simulink model "JenaFox_NCm"  (R2022a)
settings: Solver=VariableStepAuto  StartTime=0.0  StopTime=terminationConditions.stopTime  FixedStep=0.0001  MaxStep=solverParams.maxStep  RelTol=solverParams.relTol  AbsTol=solverParams.absTol
undefined symbols (not defined in the file): amplifier, c_coupling, d_coupling, g, GC, GM_h, IC, IC_v, motorHip, motorKnee, mu, offset, prop_const, smiData, terminationConditions, v, X, Y, Z
libraries: sm_lib x51, nesl_utility x46, simulink x23, simulink_extras x12, dspswit3 x2
(part 1 of 4)
settings Model: SimulationMode=accelerator  Creator=Work  LastModifiedBy=fesch
settings SolverCC: NumberNewtonIterations=2  ZeroCrossAlgorithm=Adaptive  AlgebraicLoopSolver=TrustRegion
settings DataIOCC: ExternalInput=JenaFox_NCm  FinalStateName=finalOP  SaveOperatingPoint=on  Refine=solverParams.refineFactor
settings DebuggingCC: IgnoredZcDiagnostic=none  UnconnectedInputMsg=warning  UnconnectedOutputMsg=warning  UnconnectedLineMsg=warning  SFMachineParentedDataDiag=warning  ArithmeticOperatorsInVariantConditions=warning
settings SFSimCC: SimUseLocalCustomCode=off  CustomCodeUndefinedFunction=UseInterfaceOnly
settings RTWCC: RTWUseLocalCustomCode=off  Toolchain=MinGW64 | gmake (64-bit Windows)  DLArmComputeVersion=19.05
settings ExplorerConfigSet: InternalSimMechanicsExplorerSettings="<ExplorerConfiguration><canonicalview>planar_xy</canonicalview><AnimationSetting><BasePlaybackSpeed>1.0</BasePlaybackSpeed><PlaybackSpeedFactor>0.25</PlaybackSpeedFactor></AnimationSetting><TilePanel><TileInfo><Tiles Columns=\"1\" Count=\"1\" Rows=\"1\"><Column Weight=\"1\"/><Row Weight=\"1\"/><Tile Height=\"1\" Width=\"1\" X=\"0\" Y=\"0\"/></Tiles></TileInfo><SceneInfo><SceneViewer><BGColor><R>1</R><G>1</G><B>1</B></BGColor><Camera><DoPerspective>on</DoPerspective><Position><X>0.0780946526691303905</X><Y>0.155519108041309417</Y><Z>0.5</Z></Position><Center><X>0.0780946526691303905</X><Y>0.155519108041309417</Y><Z>-0.5</Z></Center><Up><X>-9.313783918415811e-06</X><Y>0.999999999956626695</Y><Z>0</Z></Up><ViewLimDist>1</ViewLimDist><YLim>0.466307658154998583</YLim><XLim>0.934484284879756544</XLim></Camera></SceneViewer></SceneInfo></TilePanel><MechEditorPanel><Cameras><Camera><Id>Camera1</Id><Value><Name>Camera1</Name><NativeCamera><PositionTrackingFeature>JenaFox_model.Camera1.Frame1</PositionTrackingFeature><CenterTrackingFeature>JenaFox_model.Camera1.Frame1</CenterTrackingFeature><UpVectorTrackingFeature>JenaFox_model.Camera1.Frame1</UpVectorTrackingFeature><CenterTrackingOrigin>off</CenterTrackingOrigin><CenterTrackingDirection>-Z</CenterTrackingDirection><UpVectorTrackingDirection>+Y</UpVectorTrackingDirection></NativeCamera></Value></Camera></Cameras><GfxPanelCameraMap><MapElement CameraMLId=\"Camera1\" GfxPanelIndex=\"0\"/></GfxPanelCameraMap><VideoCreator><PlaybackSpeedRatio>0.25</PlaybackSpeedRatio><FrameRate>30</FrameRate><VideoFormat>Motion JPEG AVI</VideoFormat><FrameSize>auto</FrameSize></VideoCreator></MechEditorPanel></ExplorerConfiguration>"

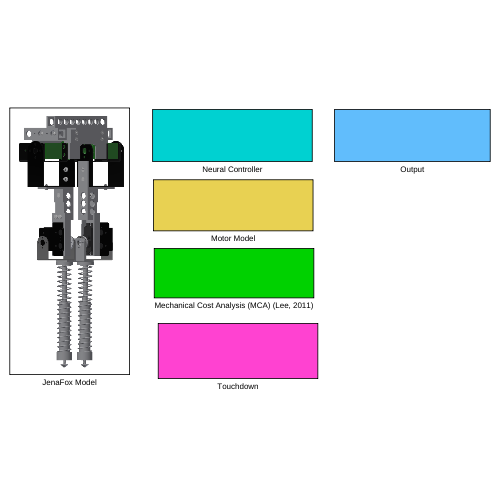
[thumbnail: Simulink's stored preview of the top-level diagram]
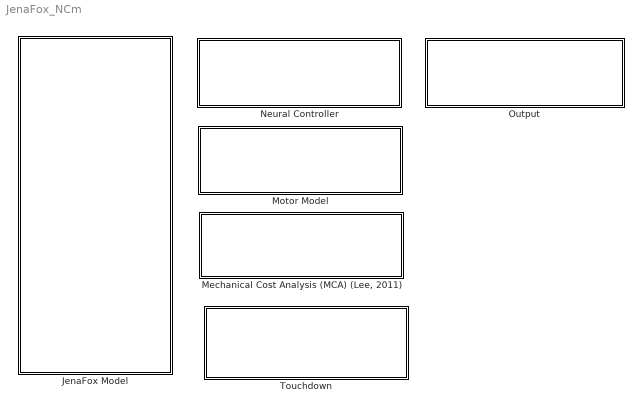
== system JenaFox_NCm ==
  JenaFox Model : Subsystem
      mask Display: image('$imagefile'); % Use "Edit Image" on toolstrip to change.
  "Mechanical Cost Analysis (MCA) (Lee, 2011)" : Subsystem
  Motor Model : Subsystem
  Neural Controller : Subsystem
  Output : Subsystem
  Touchdown : Subsystem

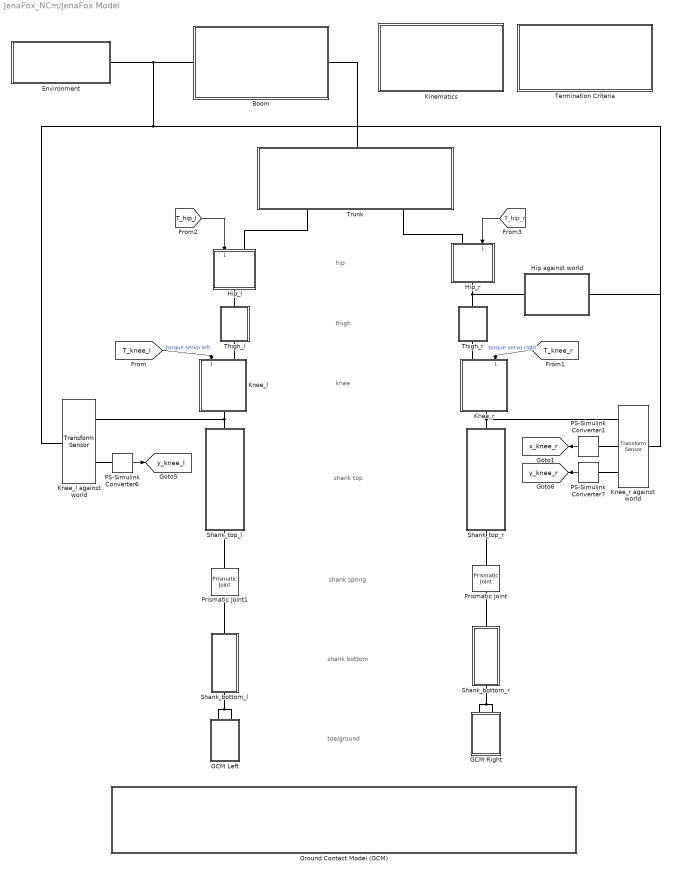
== system JenaFox_NCm/JenaFox Model ==
  note: hip
  note: thigh
  note: knee
  note: shank top
  note: shank spring
  note: shank bottom
  note: toe/ground
  Boom : Subsystem
  Environment : Subsystem
  GCM Left : Subsystem
      settings: PortSchema="{\"entries\":[{\"content\":{\"sides\":[{\"content\":{\"connectorIds\":[]},\"type\":\"ConnectorPlacement.EquallySpacedRectSide\",\"uuid\":\"717cb0e6-c62a-4e06-8591-18c3af15a403\"},{\"content\":{\"connectorIds\":[],\"side\":\"RIGHT\"},\"type\":\"ConnectorPlacement.EquallySpacedRectSide\",\"uuid\":\"b55d33af-557a-4e38-8805-fc673b8726f4\"},{\"content\":{\"connectorIds\":[\"LConn1\",\"LConn2\"],\"side\":\"TOP\"},\"type\":\"ConnectorPlacement.EquallySpacedRectSide\",\"uuid\":\"c2e40c4e-431e-4c5b-992c-f2657d397cd9\"}]},\"type\":\"ConnectorPlacement.EquallySpacedConnector\",\"uuid\":\"60787a51-cbf9-4fb7-a22c-83b01a92506b\"}],\"packageUris\":[\"http://schema.mathworks.com/mf0/Connector/R2020b\"],\"version\":\"1.0\"}"
  GCM Right : Subsystem
      settings: PortSchema="{\"entries\":[{\"content\":{\"sides\":[{\"content\":{\"connectorIds\":[]},\"type\":\"ConnectorPlacement.EquallySpacedRectSide\",\"uuid\":\"717cb0e6-c62a-4e06-8591-18c3af15a403\"},{\"content\":{\"connectorIds\":[],\"side\":\"RIGHT\"},\"type\":\"ConnectorPlacement.EquallySpacedRectSide\",\"uuid\":\"b55d33af-557a-4e38-8805-fc673b8726f4\"},{\"content\":{\"connectorIds\":[\"LConn1\",\"LConn2\"],\"side\":\"TOP\"},\"type\":\"ConnectorPlacement.EquallySpacedRectSide\",\"uuid\":\"c2e40c4e-431e-4c5b-992c-f2657d397cd9\"}]},\"type\":\"ConnectorPlacement.EquallySpacedConnector\",\"uuid\":\"60787a51-cbf9-4fb7-a22c-83b01a92506b\"}],\"packageUris\":[\"http://schema.mathworks.com/mf0/Connector/R2020b\"],\"version\":\"1.0\"}"
  Ground Contact Model (GCM) : Subsystem
  Hip against world : Subsystem
  Hip_l : Subsystem
  Hip_r : Subsystem
      settings: PortSchema="{\"entries\":[{\"content\":{\"sides\":[{\"content\":{\"connectorIds\":[\"LConn1\",\"In1\"]},\"type\":\"ConnectorPlacement.EquallySpacedRectSide\",\"uuid\":\"6727c252-b3e4-4702-a459-ab364fb8daee\"},{\"content\":{\"connectorIds\":[\"RConn1\"],\"side\":\"RIGHT\"},\"type\":\"ConnectorPlacement.EquallySpacedRectSide\",\"uuid\":\"d9cb8ba9-0a5e-46cb-8448-2d23ff2cf8a0\"},{\"content\":{\"connectorIds\":[],\"side\":\"TOP\"},\"type\":\"ConnectorPlacement.EquallySpacedRectSide\",\"uuid\":\"eb700dfb-5883-4c49-bb8c-e592edc073a0\"}]},\"type\":\"ConnectorPlacement.EquallySpacedConnector\",\"uuid\":\"4bb2fdc9-2c2e-463e-9c20-4381bcff8659\"}],\"packageUris\":[\"http://schema.mathworks.com/mf0/Connector/R2020b\"],\"version\":\"1.0\"}"
  Kinematics : Subsystem
  Knee_l : Subsystem
  Knee_l against world : sm_lib/Frames and Transforms/Transform Sensor  MeasurementFrame=World  SenseAngle=off  SenseAxis=off  SenseAngle1=off  SenseAngle2=off  SenseAngle3=off  SenseQ=off  SenseR=off  SenseOmegaX=off  SenseOmegaY=off  SenseOmegaZ=off  SenseOmega1=off  SenseOmega2=off  SenseOmega3=off  SenseQDot=off  SenseRDot=off  SenseAlphaX=off  SenseAlphaY=off  SenseAlphaZ=off  SenseAlpha1=off  SenseAlpha2=off  SenseAlpha3=off  SenseQDDot=off  SenseRDDot=off  SenseX=off  SenseY=on  SenseZ=off  SenseRad=off  SenseAzim=off  SenseDist=off  SenseInc=off  SenseXDot=off  SenseYDot=off  SenseZDot=off  SenseRadDot=off  SenseAzimDot=off  SenseDistDot=off  SenseIncDot=off  SenseXDDot=off  SenseYDDot=off  SenseZDDot=off  SenseRadDDot=off  SenseAzimDDot=off  SenseDistDDot=off  SenseIncDDot=off
  Knee_r : Subsystem
      settings: PortSchema="{\"entries\":[{\"content\":{\"sides\":[{\"content\":{\"connectorIds\":[\"LConn1\",\"In1\"]},\"type\":\"ConnectorPlacement.EquallySpacedRectSide\",\"uuid\":\"6727c252-b3e4-4702-a459-ab364fb8daee\"},{\"content\":{\"connectorIds\":[\"RConn1\"],\"side\":\"RIGHT\"},\"type\":\"ConnectorPlacement.EquallySpacedRectSide\",\"uuid\":\"d9cb8ba9-0a5e-46cb-8448-2d23ff2cf8a0\"},{\"content\":{\"connectorIds\":[],\"side\":\"TOP\"},\"type\":\"ConnectorPlacement.EquallySpacedRectSide\",\"uuid\":\"eb700dfb-5883-4c49-bb8c-e592edc073a0\"}]},\"type\":\"ConnectorPlacement.EquallySpacedConnector\",\"uuid\":\"4bb2fdc9-2c2e-463e-9c20-4381bcff8659\"}],\"packageUris\":[\"http://schema.mathworks.com/mf0/Connector/R2020b\"],\"version\":\"1.0\"}"
  Knee_r against world : sm_lib/Frames and Transforms/Transform Sensor  MeasurementFrame=World  SenseAngle=off  SenseAxis=off  SenseAngle1=off  SenseAngle2=off  SenseAngle3=off  SenseQ=off  SenseR=off  SenseOmegaX=off  SenseOmegaY=off  SenseOmegaZ=off  SenseOmega1=off  SenseOmega2=off  SenseOmega3=off  SenseQDot=off  SenseRDot=off  SenseAlphaX=off  SenseAlphaY=off  SenseAlphaZ=off  SenseAlpha1=off  SenseAlpha2=off  SenseAlpha3=off  SenseQDDot=off  SenseRDDot=off  SenseX=on  SenseY=on  SenseZ=off  SenseRad=off  SenseAzim=off  SenseDist=off  SenseInc=off  SenseXDot=off  SenseYDot=off  SenseZDot=off  SenseRadDot=off  SenseAzimDot=off  SenseDistDot=off  SenseIncDot=off  SenseXDDot=off  SenseYDDot=off  SenseZDDot=off  SenseRadDDot=off  SenseAzimDDot=off  SenseDistDDot=off  SenseIncDDot=off
  PS-Simulink Converter1 : nesl_utility/PS-Simulink Converter  PhysicalDomain=network_engine_domain  SubClassName=ps_output  LeftPortType=input  RightPortType=output  PseudoPeriodic=off  Frequencies=[]  VectorFormat=1-D array  Unit=1  AffineConversion=off
      settings: SourceProductBaseCode=SS,PW,VE
  PS-Simulink Converter6 : nesl_utility/PS-Simulink Converter  PhysicalDomain=network_engine_domain  SubClassName=ps_output  LeftPortType=input  RightPortType=output  PseudoPeriodic=off  Frequencies=[]  VectorFormat=1-D array  Unit=1  AffineConversion=off
      settings: SourceProductBaseCode=SS,PW,VE
  PS-Simulink Converter7 : nesl_utility/PS-Simulink Converter  PhysicalDomain=network_engine_domain  SubClassName=ps_output  LeftPortType=input  RightPortType=output  PseudoPeriodic=off  Frequencies=[]  VectorFormat=1-D array  Unit=1  AffineConversion=off
      settings: SourceProductBaseCode=SS,PW,VE
  Prismatic Joint : sm_lib/Joints/Prismatic Joint  JointMode=Normal  SenseConstraintForce=off  SenseConstraintForceX=off  SenseConstraintForceY=off  SenseConstraintForceZ=off  SenseConstraintTorque=off  SenseConstraintTorqueX=off  SenseConstraintTorqueY=off  SenseConstraintTorqueZ=off  SenseTotalForce=off  SenseTotalForceX=off  SenseTotalForceY=off  SenseTotalForceZ=off  SenseTotalTorque=off  SenseTotalTorqueX=off  SenseTotalTorqueY=off  SenseTotalTorqueZ=off  CompositeWrenchDir=FollowerOnBase  CompositeWrenchFrame=BaseFrame  EquilibriumPosition=0  EquilibriumPositionUnits=m  SpringStiffness=springAnkle.c_r  SpringStiffnessUnits=N/m  DampingCoefficient=damperAnkle.r  DampingCoefficientUnits=N/(m/s)  TorqueActuationMode=NoTorque  MotionActuationMode=ComputedMotion  SensePosition=off  SenseVelocity=off  SenseAcceleration=off  SenseTorqueForce=off  SenseLowerLimitTorqueForce=off  SenseUpperLimitTorqueForce=off  LowerLimitSpecify=off  LowerLimitBound=-1  LowerLimitBoundUnits=m  LowerLimitStiffness=1e6  LowerLimitStiffnessUnits=N/m  LowerLimitDamping=1e3  LowerLimitDampingUnits=N/(m/s)  LowerLimitTransitionRegionWidth=1e-4  LowerLimitTransitionRegionWidthUnits=m  UpperLimitSpecify=on  UpperLimitBound=0  UpperLimitBoundUnits=m  UpperLimitStiffness=1e6  UpperLimitStiffnessUnits=N/m  UpperLimitDamping=1e3  UpperLimitDampingUnits=N/(m/s)  UpperLimitTransitionRegionWidth=1e-4  UpperLimitTransitionRegionWidthUnits=m  PositionTargetSpecify=off  PositionTargetPriority=High  PositionTargetValue=0  PositionTargetValueUnits=m  VelocityTargetSpecify=off  VelocityTargetPriority=High  VelocityTargetValue=0  VelocityTargetValueUnits=m/s
  Prismatic Joint1 : sm_lib/Joints/Prismatic Joint  JointMode=Normal  SenseConstraintForce=off  SenseConstraintForceX=off  SenseConstraintForceY=off  SenseConstraintForceZ=off  SenseConstraintTorque=off  SenseConstraintTorqueX=off  SenseConstraintTorqueY=off  SenseConstraintTorqueZ=off  SenseTotalForce=off  SenseTotalForceX=off  SenseTotalForceY=off  SenseTotalForceZ=off  SenseTotalTorque=off  SenseTotalTorqueX=off  SenseTotalTorqueY=off  SenseTotalTorqueZ=off  CompositeWrenchDir=FollowerOnBase  CompositeWrenchFrame=BaseFrame  EquilibriumPosition=0  EquilibriumPositionUnits=m  SpringStiffness=springAnkle.c_l  SpringStiffnessUnits=N/m  DampingCoefficient=damperAnkle.l  DampingCoefficientUnits=N/(m/s)  TorqueActuationMode=NoTorque  MotionActuationMode=ComputedMotion  SensePosition=off  SenseVelocity=off  SenseAcceleration=off  SenseTorqueForce=off  SenseLowerLimitTorqueForce=off  SenseUpperLimitTorqueForce=off  LowerLimitSpecify=off  LowerLimitBound=-1  LowerLimitBoundUnits=m  LowerLimitStiffness=1e6  LowerLimitStiffnessUnits=N/m  LowerLimitDamping=1e3  LowerLimitDampingUnits=N/(m/s)  LowerLimitTransitionRegionWidth=1e-4  LowerLimitTransitionRegionWidthUnits=m  UpperLimitSpecify=on  UpperLimitBound=0  UpperLimitBoundUnits=m  UpperLimitStiffness=1e6  UpperLimitStiffnessUnits=N/m  UpperLimitDamping=1e3  UpperLimitDampingUnits=N/(m/s)  UpperLimitTransitionRegionWidth=1e-4  UpperLimitTransitionRegionWidthUnits=m  PositionTargetSpecify=off  PositionTargetPriority=High  PositionTargetValue=0  PositionTargetValueUnits=m  VelocityTargetSpecify=off  VelocityTargetPriority=High  VelocityTargetValue=0  VelocityTargetValueUnits=m/s
  Shank_bottom_l : Subsystem
  Shank_bottom_r : Subsystem
  Shank_top_l : Subsystem
  Shank_top_r : Subsystem
  Termination Criteria : Subsystem
  Thigh_l : Subsystem
  Thigh_r : Subsystem
  Trunk : Subsystem
  tag scope: x_knee_r=global, y_knee_l=global, y_knee_r=global
  wires:
  [T_knee_l] -> Knee_l/1(Left torque)  "torque servo left"
  [T_knee_r] -> Knee_r/1(Right torque)  "torque servo right"
  [T_hip_l] -> Hip_l/1(Left torque)
  [T_hip_r] -> Hip_r/1(Right torque)
  PS-Simulink Converter6/1 -> [y_knee_l]
  PS-Simulink Converter7/1 -> [y_knee_r]
  PS-Simulink Converter1/1 -> [x_knee_r]
  connections:
  Knee_r/RConn1 -- Knee_r against world/RConn1 -- Shank_top_r/LConn1
  Knee_r/LConn1 -- Thigh_r/RConn1
  Prismatic Joint1/LConn1 -- Shank_bottom_l/LConn1
  Hip_l/RConn1 -- Thigh_l/LConn1
  GCM Right/LConn2 -- GCM Right/LConn1 -- Shank_bottom_r/RConn1
  Prismatic Joint/RConn1 -- Shank_top_r/RConn1
  Knee_l/LConn1 -- Thigh_l/RConn1
  Prismatic Joint1/RConn1 -- Shank_top_l/RConn1
  Prismatic Joint/LConn1 -- Shank_bottom_r/LConn1
  GCM Left/LConn2 -- GCM Left/LConn1 -- Shank_bottom_l/RConn1
  Hip_r/LConn1 -- Trunk/RConn2
  Shank_top_l/LConn1 -- Knee_l against world/RConn1 -- Knee_l/RConn1
  Environment/RConn1 -- Hip against world/LConn1 -- Knee_r against world/LConn1 -- Knee_l against world/LConn1 -- Boom/LConn1
  Boom/RConn1 -- Trunk/LConn1
  Knee_l against world/RConn2 -- PS-Simulink Converter6/LConn1
  Hip_l/LConn1 -- Trunk/RConn1
  Hip_r/RConn1 -- Hip against world/RConn1 -- Thigh_r/LConn1
  Knee_r against world/RConn3 -- PS-Simulink Converter7/LConn1
  PS-Simulink Converter1/LConn1 -- Knee_r against world/RConn2

== system JenaFox_NCm/Mechanical Cost Analysis (MCA) (Lee, 2011) ==
  Bus Creator : BusCreator  Inputs=8
  Bus Selector : BusSelector  OutputSignals=x_com,y_com,dx_com,dy_com,vphi_com_world
  Bus Selector2 : BusSelector  OutputSignals=x_hip,y_hip,dx_hip,dy_hip
  Constant : Constant  Value=prop_const
  Constant1 : Constant  Value=offset
  Demux : Demux  Outputs=2
  Mechanical Cost Analysis (MCA) : MATLAB Function  TreatAsAtomicUnit=on
  Mux{,1..2,4} (4 alike) : Mux  Inputs=2
  tag scope: mechanical_cost_analysis=global
  wires:
  [hip_kinematics] -> Bus Selector2/1
  Bus Selector2/3 -> Mux2/1  "<dx_hip>"
  Mux2/1 -> Mechanical Cost Analysis (MCA)/6(V_hip)  "velocity vector hip"
  Bus Creator/1 -> [mechanical_cost_analysis]
  [com_kinematics] -> Bus Selector/1
  Bus Selector2/4 -> Mux2/2  "<dy_hip>"
  [GRF] -> Mechanical Cost Analysis (MCA)/1(GRF)  "force vector"
  Bus Selector/4 -> Mux/2  "<dy_com>"
  Bus Selector/3 -> Mux/1  "<dx_com>"
  Bus Selector/1 -> Mux4/1  "<x_com>"
  Bus Selector/2 -> Mux4/2  "<y_com>"
  Mux4/1 -> Mechanical Cost Analysis (MCA)/2(origin_com)
  Bus Selector2/1 -> Mux1/1  "<x_hip>"
  Bus Selector2/2 -> Mux1/2  "<y_hip>"
  Mux1/1 -> Mechanical Cost Analysis (MCA)/5(origin_hip)
  Mechanical Cost Analysis (MCA)/1(theta_com) -> Bus Creator/1  "theta_com"
  Mux/1 -> Mechanical Cost Analysis (MCA)/3(V_com)  "velocity vector com"
  Constant1/1 -> Mechanical Cost Analysis (MCA)/8(offset)
  Mechanical Cost Analysis (MCA)/2(lambda_com) -> Bus Creator/2  "lambda_com"
  Bus Selector/5 -> Mechanical Cost Analysis (MCA)/4(vphi_com)  "<vphi_com_world>"
  Mechanical Cost Analysis (MCA)/3(lambda_hip) -> Bus Creator/3  "lambda_hip"
  Mechanical Cost Analysis (MCA)/6(V_proj) -> Demux/1  "V_proj"
  Mechanical Cost Analysis (MCA)/4(lambda_proj) -> Bus Creator/4  "lambda_proj"
  Mechanical Cost Analysis (MCA)/5(phi_com) -> Bus Creator/5  "phi_com"
  Demux/1 -> Bus Creator/6  "V_proj_x"
  Demux/2 -> Bus Creator/7  "V_proj_y"
  Mechanical Cost Analysis (MCA)/7(AEA) -> Bus Creator/8  "AEA"
  Constant/1 -> Mechanical Cost Analysis (MCA)/7(prop_const)

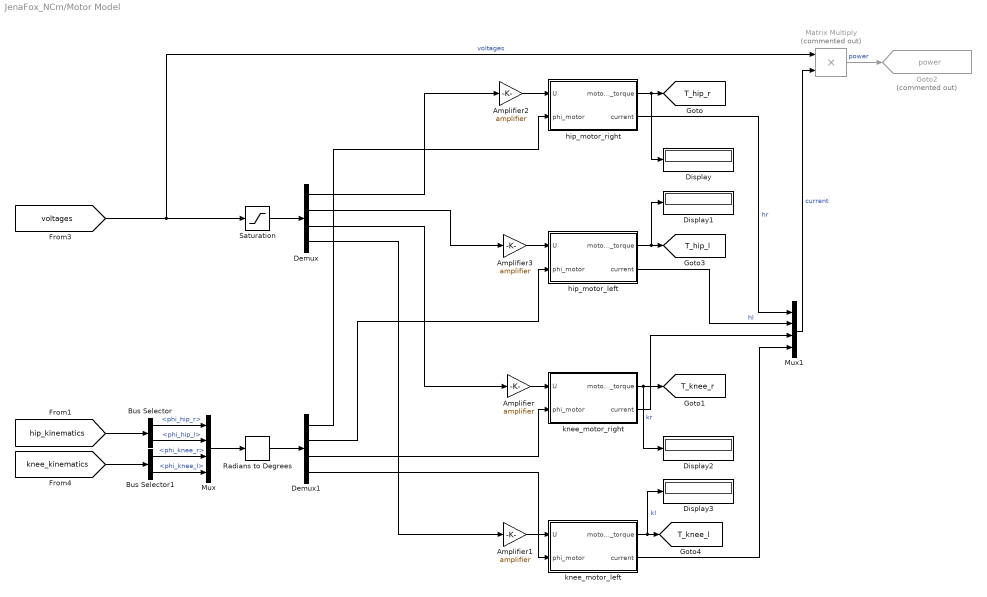
== system JenaFox_NCm/Motor Model ==
  Amplifier{,1..3} (4 alike) : Gain  Gain=amplifier
  Bus Selector : BusSelector  OutputSignals=phi_hip_r,phi_hip_l
  Bus Selector1 : BusSelector  OutputSignals=phi_knee_r,phi_knee_l
  Demux : Demux
  Demux1 : Demux
  Display{,1..3} (4 alike) : Display
  Goto2 : Goto  Commented=on  GotoTag=power  TagVisibility=global
  Matrix Multiply : Product  Commented=on
  Mux : Mux
  Mux1 : Mux
  Radians to Degrees : simulink_extras/Transformations/Radians to Degrees
  Saturation : Saturate  UpperLimit=5  LowerLimit=-5
  hip_motor_left : Subsystem  mask(Hip Motor){IC_phi_motor_hip=IC.motor.hip_l}
      mask prompts: IC_phi_motor_hip "Initial position"
  hip_motor_right : Subsystem  mask(Hip Motor){IC_phi_motor_hip=IC.motor.hip_r}
      mask prompts: IC_phi_motor_hip "Initial position"
  knee_motor_left : Subsystem  mask{IC_phi_motor_knee=IC.motor.knee_l}
      mask prompts: IC_phi_motor_knee "Initial motor position"
  knee_motor_right : Subsystem  mask{IC_phi_motor_knee=IC.motor.knee_r}
      mask prompts: IC_phi_motor_knee "Initial motor position"
  tag scope: T_hip_l=global, T_hip_r=global, T_knee_l=global, T_knee_r=global
  wires:
  Amplifier/1 -> knee_motor_right/1(U)
  knee_motor_left/1(motor_torque) -> Display3/1, [T_knee_l]  "kl"
  Saturation/1 -> Demux/1
  Amplifier1/1 -> knee_motor_left/1(U)
  Demux/1 -> Amplifier2/1
  knee_motor_right/2(current) -> Mux1/3
  Amplifier2/1 -> hip_motor_right/1(U)
  Demux1/4 -> knee_motor_left/2(phi_motor)
  hip_motor_left/1(motor_torque) -> Display1/1, [T_hip_l]
  hip_motor_right/1(motor_torque) -> Display/1, [T_hip_r]
  knee_motor_right/1(motor_torque) -> [T_knee_r], Display2/1  "kr"
  hip_motor_right/2(current) -> Mux1/1  "hr"
  Mux1/1 -> Matrix Multiply/2  "current"
  Amplifier3/1 -> hip_motor_left/1(U)
  Demux/2 -> Amplifier3/1
  Demux1/1 -> hip_motor_right/2(phi_motor)
  Demux1/2 -> hip_motor_left/2(phi_motor)
  hip_motor_left/2(current) -> Mux1/2  "hl"
  Matrix Multiply/1 -> Goto2/1  "power"
  Demux1/3 -> knee_motor_right/2(phi_motor)
  Demux/4 -> Amplifier1/1
  Demux/3 -> Amplifier/1
  knee_motor_left/2(current) -> Mux1/4
  Bus Selector1/1 -> Mux/3  "<phi_knee_r>"
  [hip_kinematics] -> Bus Selector/1
  Bus Selector1/2 -> Mux/4  "<phi_knee_l>"
  Bus Selector/1 -> Mux/1  "<phi_hip_r>"
  [knee_kinematics] -> Bus Selector1/1
  Mux/1 -> Radians to Degrees/1
  Bus Selector/2 -> Mux/2  "<phi_hip_l>"
  [voltages] -> Saturation/1, Matrix Multiply/1  "voltages"
  Radians to Degrees/1 -> Demux1/1

== system JenaFox_NCm/Neural Controller ==
  Bus Selector : BusSelector  OutputSignals=phi_hip_r,phi_hip_l
  Bus Selector1 : BusSelector  OutputSignals=phi_knee_r,phi_knee_l
  Bus Selector2 : BusSelector  OutputSignals=AEA
  Clock : Clock
  Constant : Constant  Value=GM_h
  Memory : Memory  InitialCondition=[0 0;0 0;0 0;0 0;0 0]
  Mux : Mux
  Neural Network Based Controller : MATLAB Function  TreatAsAtomicUnit=on  SystemSampleTime=1e-3
  Radians to Degrees : simulink_extras/Transformations/Radians to Degrees
  tag scope: voltages=global
  wires:
  Neural Network Based Controller/1(U) -> [voltages]
  [ground_contact] -> Neural Network Based Controller/3(GC)
  Mux/1 -> Radians to Degrees/1
  Memory/1 -> Neural Network Based Controller/6("y_old ")
  Neural Network Based Controller/2(y_old) -> Memory/1
  Clock/1 -> Neural Network Based Controller/1(t)
  [hip_kinematics] -> Bus Selector/1
  [knee_kinematics] -> Bus Selector1/1
  Bus Selector1/1 -> Mux/3  "<phi_knee_r>"
  Bus Selector1/2 -> Mux/4  "<phi_knee_l>"
  Bus Selector/2 -> Mux/2  "<phi_hip_l>"
  Bus Selector/1 -> Mux/1  "<phi_hip_r>"
  [mechanical_cost_analysis] -> Bus Selector2/1
  Constant/1 -> Neural Network Based Controller/5(GM_h)
  Radians to Degrees/1 -> Neural Network Based Controller/2(phi)
  Bus Selector2/1 -> Neural Network Based Controller/4(AEA)  "<AEA>"

== system JenaFox_NCm/Output ==
  Bus Creator : BusCreator  Inputs=1
  To Workspace : ToWorkspace  VariableName=touchdown  SaveFormat=Timeseries  SampleTime=-1
  To Workspace1 : ToWorkspace  VariableName=com_kinematics  SaveFormat=Timeseries  SampleTime=-1
  To Workspace2 : ToWorkspace  VariableName=output  SaveFormat=Timeseries  SampleTime=-1
  To Workspace3 : ToWorkspace  VariableName=ground_contact_model  SaveFormat=Timeseries  SampleTime=-1
  To Workspace6 : ToWorkspace  VariableName=toe_kinematics  SaveFormat=Timeseries  SampleTime=-1
  To Workspace7 : ToWorkspace  VariableName=hip_kinematics  SaveFormat=Timeseries  SampleTime=-1
  To Workspace8 : ToWorkspace  VariableName=knee_kinematics  SaveFormat=Timeseries  SampleTime=-1
  To Workspace9 : ToWorkspace  VariableName=mechanical_cost_analysis  SaveFormat=Timeseries  SampleTime=-1
  wires:
  [com_kinematics] -> To Workspace1/1
  [mechanical_cost_analysis] -> To Workspace9/1
  [touchdown] -> To Workspace/1
  [hip_kinematics] -> To Workspace7/1
  [knee_kinematics] -> To Workspace8/1
  [status] -> Bus Creator/1  "status"
  [toe_kinematics] -> To Workspace6/1
  [ground_contact_model] -> To Workspace3/1
  Bus Creator/1 -> To Workspace2/1

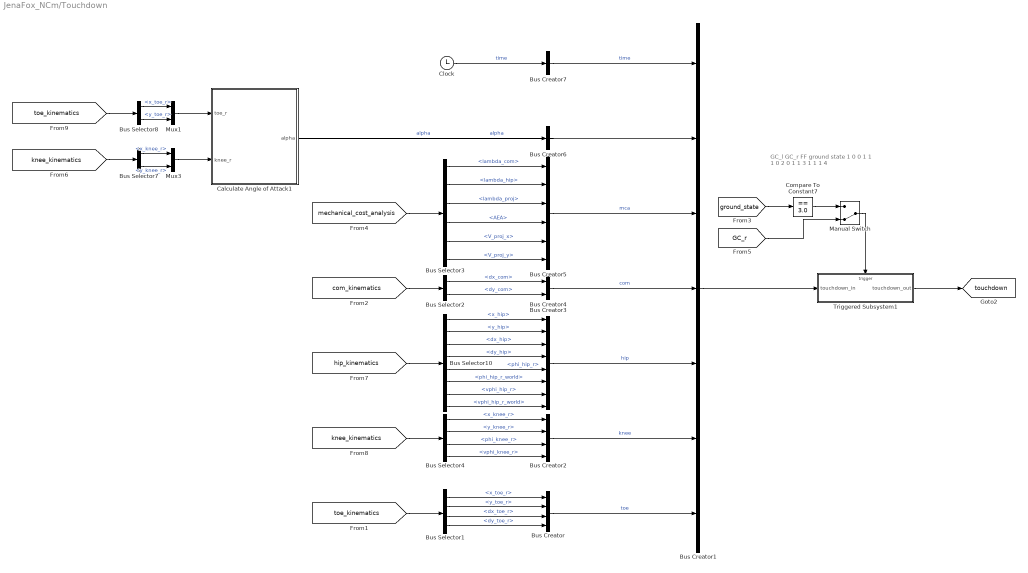
== system JenaFox_NCm/Touchdown ==
  note: GC_l   GC_r   FF   ground state
      | 1         0         0       1
      | 1         1         0       2
      | 0         1         1       3
      | 1         1         1       4
  Bus Creator : BusCreator  Inputs=4
  Bus Creator1 : BusCreator  Inputs=7
  Bus Creator2 : BusCreator  Inputs=4
  Bus Creator3 : BusCreator  Inputs=8
  Bus Creator4 : BusCreator  Inputs=2
  Bus Creator5 : BusCreator  Inputs=6
  Bus Creator6 : BusCreator  Inputs=1
  Bus Creator7 : BusCreator  Inputs=1
  Bus Selector1 : BusSelector  OutputSignals=x_toe_r,y_toe_r,dx_toe_r,dy_toe_r
  Bus Selector10 : BusSelector  OutputSignals=x_hip,y_hip,dx_hip,dy_hip,phi_hip_r,phi_hip_r_world,vphi_hip_r,vphi_hip_r_world
  Bus Selector2 : BusSelector  OutputSignals=dx_com,dy_com
  Bus Selector3 : BusSelector  OutputSignals=lambda_com,lambda_hip,lambda_proj,AEA,V_proj_x,V_proj_y
  Bus Selector4 : BusSelector  OutputSignals=x_knee_r,y_knee_r,phi_knee_r,vphi_knee_r
  Bus Selector7 : BusSelector  OutputSignals=x_knee_r,y_knee_r
  Bus Selector8 : BusSelector  OutputSignals=x_toe_r,y_toe_r
  Calculate Angle of Attack1 : MATLAB Function  TreatAsAtomicUnit=on
  Clock : Clock
  Compare To Constant7 : simulink/Logic and Bit Operations/Compare To Constant  relop===  const=3.0  OutDataTypeStr=boolean
  Manual Switch : ManualSwitch  CurrentSetting=0
  Mux1 : Mux  Inputs=2
  Mux3 : Mux  Inputs=2
  Triggered Subsystem1 : Subsystem  TreatAsAtomicUnit=on
  tag scope: touchdown=global
  wires:
  Clock/1 -> Bus Creator7/1  "time"
  [knee_kinematics] -> Bus Selector4/1
  [hip_kinematics] -> Bus Selector10/1
  [com_kinematics] -> Bus Selector2/1
  [ground_state] -> Compare To Constant7/1
  [mechanical_cost_analysis] -> Bus Selector3/1
  [toe_kinematics] -> Bus Selector1/1
  Bus Creator1/1 -> Triggered Subsystem1/1(touchdown_in)
  Triggered Subsystem1/1(touchdown_out) -> [touchdown]
  Compare To Constant7/1 -> Manual Switch/1
  Manual Switch/1 -> Triggered Subsystem1/Trigger
  [GC_r] -> Manual Switch/2
  [toe_kinematics] -> Bus Selector8/1
  Mux1/1 -> Calculate Angle of Attack1/1(toe_r)
  Bus Selector8/1 -> Mux1/1  "<x_toe_r>"
  Bus Selector8/2 -> Mux1/2  "<y_toe_r>"
  Mux3/1 -> Calculate Angle of Attack1/2(knee_r)
  [knee_kinematics] -> Bus Selector7/1
  Bus Selector7/1 -> Mux3/1  "<x_knee_r>"
  Bus Selector7/2 -> Mux3/2  "<y_knee_r>"
  Calculate Angle of Attack1/1(alpha) -> Bus Creator6/1  "alpha"
  Bus Selector10/8 -> Bus Creator3/8  "<vphi_hip_r_world>"
  Bus Selector10/7 -> Bus Creator3/7  "<vphi_hip_r>"
  Bus Selector10/6 -> Bus Creator3/6  "<phi_hip_r_world>"
  Bus Selector10/5 -> Bus Creator3/5  "<phi_hip_r>"
  Bus Selector10/4 -> Bus Creator3/4  "<dy_hip>"
  Bus Selector10/3 -> Bus Creator3/3  "<dx_hip>"
  Bus Selector10/2 -> Bus Creator3/2  "<y_hip>"
  Bus Selector10/1 -> Bus Creator3/1  "<x_hip>"
  Bus Selector2/1 -> Bus Creator4/1  "<dx_com>"
  Bus Selector2/2 -> Bus Creator4/2  "<dy_com>"
  Bus Selector3/1 -> Bus Creator5/1  "<lambda_com>"
  Bus Selector3/2 -> Bus Creator5/2  "<lambda_hip>"
  Bus Selector3/3 -> Bus Creator5/3  "<lambda_proj>"
  Bus Selector3/4 -> Bus Creator5/4  "<AEA>"
  Bus Selector3/5 -> Bus Creator5/5  "<V_proj_x>"
  Bus Selector3/6 -> Bus Creator5/6  "<V_proj_y>"
  Bus Creator5/1 -> Bus Creator1/3  "mca"
  Bus Creator4/1 -> Bus Creator1/4  "com"
  Bus Creator3/1 -> Bus Creator1/5  "hip"
  Bus Creator/1 -> Bus Creator1/7  "toe"
  Bus Creator2/1 -> Bus Creator1/6  "knee"
  Bus Creator6/1 -> Bus Creator1/2  "alpha"
  Bus Creator7/1 -> Bus Creator1/1  "time"
  Bus Selector4/4 -> Bus Creator2/4  "<vphi_knee_r>"
  Bus Selector4/3 -> Bus Creator2/3  "<phi_knee_r>"
  Bus Selector4/2 -> Bus Creator2/2  "<y_knee_r>"
  Bus Selector4/1 -> Bus Creator2/1  "<x_knee_r>"
  Bus Selector1/1 -> Bus Creator/1  "<x_toe_r>"
  Bus Selector1/3 -> Bus Creator/3  "<dx_toe_r>"
  Bus Selector1/2 -> Bus Creator/2  "<y_toe_r>"
  Bus Selector1/4 -> Bus Creator/4  "<dy_toe_r>"

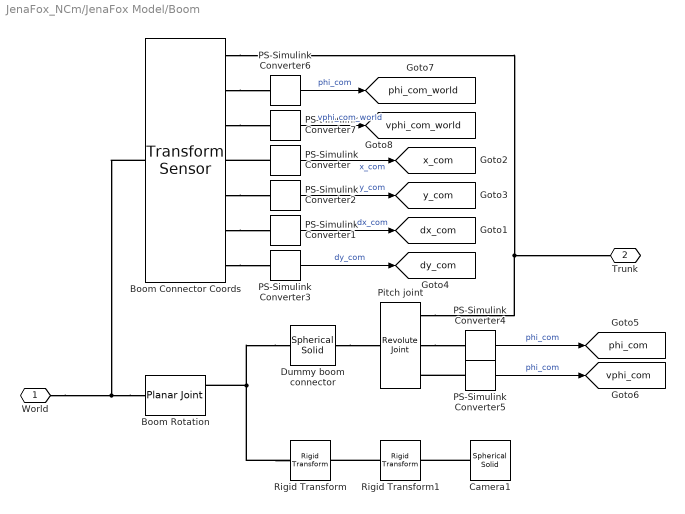
== system JenaFox_NCm/JenaFox Model/Boom ==
  Boom Connector Coords : sm_lib/Frames and Transforms/Transform Sensor  MeasurementFrame=World  SenseAngle=on  SenseAxis=off  SenseAngle1=off  SenseAngle2=off  SenseAngle3=off  SenseQ=off  SenseR=off  SenseOmegaX=off  SenseOmegaY=off  SenseOmegaZ=on  SenseOmega1=off  SenseOmega2=off  SenseOmega3=off  SenseQDot=off  SenseRDot=off  SenseAlphaX=off  SenseAlphaY=off  SenseAlphaZ=off  SenseAlpha1=off  SenseAlpha2=off  SenseAlpha3=off  SenseQDDot=off  SenseRDDot=off  SenseX=on  SenseY=on  SenseZ=off  SenseRad=off  SenseAzim=off  SenseDist=off  SenseInc=off  SenseXDot=on  SenseYDot=on  SenseZDot=off  SenseRadDot=off  SenseAzimDot=off  SenseDistDot=off  SenseIncDot=off  SenseXDDot=off  SenseYDDot=off  SenseZDDot=off  SenseRadDDot=off  SenseAzimDDot=off  SenseDistDDot=off  SenseIncDDot=off
  Boom Rotation : sm_lib/Joints/Planar Joint  JointMode=Normal  SenseConstraintForce=off  SenseConstraintForceX=off  SenseConstraintForceY=off  SenseConstraintForceZ=off  SenseConstraintTorque=off  SenseConstraintTorqueX=off  SenseConstraintTorqueY=off  SenseConstraintTorqueZ=off  SenseTotalForce=off  SenseTotalForceX=off  SenseTotalForceY=off  SenseTotalForceZ=off  SenseTotalTorque=off  SenseTotalTorqueX=off  SenseTotalTorqueY=off  SenseTotalTorqueZ=off  CompositeWrenchDir=FollowerOnBase  CompositeWrenchFrame=BaseFrame  PxEquilibriumPosition=0  PxEquilibriumPositionUnits=m  PxSpringStiffness=0  PxSpringStiffnessUnits=N/m  PxDampingCoefficient=0  PxDampingCoefficientUnits=N/(m/s)  PxTorqueActuationMode=NoTorque  PxMotionActuationMode=ComputedMotion  PxSensePosition=off  PxSenseVelocity=off  PxSenseAcceleration=off  PxSenseTorqueForce=off  PxSenseLowerLimitTorqueForce=off  PxSenseUpperLimitTorqueForce=off  PxLowerLimitSpecify=off  PxLowerLimitBound=-1  PxLowerLimitBoundUnits=m  PxLowerLimitStiffness=1e6  PxLowerLimitStiffnessUnits=N/m  PxLowerLimitDamping=1e3  PxLowerLimitDampingUnits=N/(m/s)  PxLowerLimitTransitionRegionWidth=1e-4  PxLowerLimitTransitionRegionWidthUnits=m  PxUpperLimitSpecify=off  PxUpperLimitBound=1  PxUpperLimitBoundUnits=m  PxUpperLimitStiffness=1e6  PxUpperLimitStiffnessUnits=N/m  PxUpperLimitDamping=1e3  PxUpperLimitDampingUnits=N/(m/s)  PxUpperLimitTransitionRegionWidth=1e-4  PxUpperLimitTransitionRegionWidthUnits=m  PxPositionTargetSpecify=off  PxPositionTargetPriority=High  PxPositionTargetValue=0  PxPositionTargetValueUnits=m  PxVelocityTargetSpecify=on  PxVelocityTargetPriority=High  PxVelocityTargetValue=IC.dx_com  PxVelocityTargetValueUnits=m/s  PyEquilibriumPosition=IC.y_com  PyEquilibriumPositionUnits=m  PySpringStiffness=0  PySpringStiffnessUnits=N/m  PyDampingCoefficient=0  PyDampingCoefficientUnits=N/(m/s)  PyTorqueActuationMode=NoTorque  PyMotionActuationMode=ComputedMotion  PySensePosition=off  PySenseVelocity=off  PySenseAcceleration=off  PySenseTorqueForce=off  PySenseLowerLimitTorqueForce=off  PySenseUpperLimitTorqueForce=off  PyLowerLimitSpecify=off  PyLowerLimitBound=-1  PyLowerLimitBoundUnits=m  PyLowerLimitStiffness=1e6  PyLowerLimitStiffnessUnits=N/m  PyLowerLimitDamping=1e3  PyLowerLimitDampingUnits=N/(m/s)  PyLowerLimitTransitionRegionWidth=1e-4  PyLowerLimitTransitionRegionWidthUnits=m  PyUpperLimitSpecify=off  PyUpperLimitBound=1  PyUpperLimitBoundUnits=m  PyUpperLimitStiffness=1e6  PyUpperLimitStiffnessUnits=N/m  PyUpperLimitDamping=1e3  PyUpperLimitDampingUnits=N/(m/s)  PyUpperLimitTransitionRegionWidth=1e-4  PyUpperLimitTransitionRegionWidthUnits=m  PyPositionTargetSpecify=on  PyPositionTargetPriority=High  PyPositionTargetValue=IC.y_com  PyPositionTargetValueUnits=m  PyVelocityTargetSpecify=on  PyVelocityTargetPriority=High  PyVelocityTargetValue=IC.dy_com  PyVelocityTargetValueUnits=m/s  RzEquilibriumPosition=0  RzEquilibriumPositionUnits=deg  RzSpringStiffness=500  RzSpringStiffnessUnits=N*m/deg  RzDampingCoefficient=500  RzDampingCoefficientUnits=N*m/(deg/s)  RzTorqueActuationMode=NoTorque  RzMotionActuationMode=ComputedMotion  RzSensePosition=on  RzSenseVelocity=off  RzSenseAcceleration=off  RzSenseTorqueForce=off  RzSenseLowerLimitTorqueForce=off  RzSenseUpperLimitTorqueForce=off  RzLowerLimitSpecify=off  RzLowerLimitBound=-90  RzLowerLimitBoundUnits=deg  RzLowerLimitStiffness=1e4  RzLowerLimitStiffnessUnits=N*m/deg  RzLowerLimitDamping=10  RzLowerLimitDampingUnits=N*m/(deg/s)  RzLowerLimitTransitionRegionWidth=0.1  RzLowerLimitTransitionRegionWidthUnits=deg  RzUpperLimitSpecify=off  RzUpperLimitBound=90  RzUpperLimitBoundUnits=deg  RzUpperLimitStiffness=1e4  RzUpperLimitStiffnessUnits=N*m/deg  RzUpperLimitDamping=10  RzUpperLimitDampingUnits=N*m/(deg/s)  RzUpperLimitTransitionRegionWidth=0.1  RzUpperLimitTransitionRegionWidthUnits=deg  RzPositionTargetSpecify=on  RzPositionTargetPriority=High  RzPositionTargetValue=0  RzPositionTargetValueUnits=deg  RzVelocityTargetSpecify=on  RzVelocityTargetPriority=High  RzVelocityTargetValue=0  RzVelocityTargetValueUnits=deg/s
  Camera1 : sm_lib/Body Elements/Spherical Solid  GraphicAmbientColor=[0.15 0.15 0.15 1.0]  BasedOnType=Density  CenterOfMass=[0 0 0]  CenterOfMassUnits=m  GraphicDiffuseColor=[0.5 0.5 0.5]  Density=1000  DensityUnits=kg/m^3  DoExposeReferenceFrame=off  GraphicEmissiveColor=[0.0 0.0 0.0 1.0]  ExportEntireGeometry=off  SerializedExposedGeometries=<ExposedGeometries/>  SerializedFrames=<Frames><Frame><Id>Frame1</Id><Value><Name>Frame</Name><Origin><Source>CenterOfMassFrame</Source><FeatureName></FeatureName></Origin><PrimaryAxis><DefinedDirection>+Z</DefinedDirection><Source>ReferenceFrame</Source><SourceDirection>+Z</SourceDirection><FeatureName></FeatureName></PrimaryAxis><SecondaryAxis><DefinedDirection>+X</DefinedDirection><Source>ReferenceFrame</Source><SourceDirection>+X</SourceDirection><FeatureName></FeatureName></SecondaryAxis></Value></Frame></Frames>  MarkerShape=Sphere  MarkerSize=10  GraphicType=FromGeometry  InertiaType=Custom  Mass=0  MassUnits=kg  MomentsOfInertia=[0 0 0]  MomentsOfInertiaUnits=kg*m^2  GraphicOpacity=1.0  ProductsOfInertia=[0 0 0]  ProductsOfInertiaUnits=kg*m^2  GraphicShininess=75  GraphicSpecularColor=[0.5 0.5 0.5 1.0]  SphereRadius=1e-6  SphereRadiusUnits=m  GraphicVisPropType=SimpleVisualProperties
  Dummy boom connector : sm_lib/Body Elements/Spherical Solid  GraphicAmbientColor=[0.15 0.15 0.15 1.0]  BasedOnType=Density  CenterOfMass=[0 0 0]  CenterOfMassUnits=m  GraphicDiffuseColor=[0.5 0.5 0.5]  Density=0.00001  DensityUnits=kg/m^3  DoExposeReferenceFrame=off  GraphicEmissiveColor=[0.0 0.0 0.0 1.0]  ExportEntireGeometry=off  SerializedExposedGeometries=<ExposedGeometries/>  SerializedFrames=<Frames><Frame><Id>Frame1</Id><Value><Name>O</Name><Origin><Source>ReferenceFrame</Source><FeatureName></FeatureName></Origin><PrimaryAxis><DefinedDirection>+Z</DefinedDirection><Source>ReferenceFrame</Source><SourceDirection>+Z</SourceDirection><FeatureName></FeatureName></PrimaryAxis><SecondaryAxis><DefinedDirection>+X</DefinedDirection><Source>ReferenceFrame</Source><SourceDirection>+X</SourceDirection><FeatureName></FeatureName></SecondaryAxis></Value></Frame><Frame><Id>Frame2</Id><Value><Name>E</Name><Origin><Source>ReferenceFrame</Source><FeatureName></FeatureName></Origin><PrimaryAxis><DefinedDirection>+Z</DefinedDirection><Source>ReferenceFrame</Source><SourceDirection>+Z</SourceDirection><FeatureName></FeatureName></PrimaryAxis><SecondaryAxis><DefinedDirection>+X</DefinedDirection><Source>ReferenceFrame</Source><SourceDirection>+X</SourceDirection><FeatureName></FeatureName></SecondaryAxis></Value></Frame></Frames>  MarkerShape=Sphere  MarkerSize=10  GraphicType=None  InertiaType=CalculateFromGeometry  Mass=0.0001  MassUnits=kg  MomentsOfInertia=[1 1 1]*0.001  MomentsOfInertiaUnits=kg*m^2  GraphicOpacity=1.0  ProductsOfInertia=[0 0 0]  ProductsOfInertiaUnits=kg*m^2  GraphicShininess=75  GraphicSpecularColor=[0.5 0.5 0.5 1.0]  SphereRadius=1  SphereRadiusUnits=cm  GraphicVisPropType=SimpleVisualProperties
  PS-Simulink Converter{,1..7} (8 alike) : nesl_utility/PS-Simulink Converter  PhysicalDomain=network_engine_domain  SubClassName=ps_output  LeftPortType=input  RightPortType=output  PseudoPeriodic=off  Frequencies=[]  VectorFormat=1-D array  Unit=1  AffineConversion=off
      settings: SourceProductBaseCode=SS,PW,VE
  Pitch joint : sm_lib/Joints/Revolute Joint  JointMode=Normal  SenseConstraintForce=off  SenseConstraintForceX=off  SenseConstraintForceY=off  SenseConstraintForceZ=off  SenseConstraintTorque=off  SenseConstraintTorqueX=off  SenseConstraintTorqueY=off  SenseConstraintTorqueZ=off  SenseTotalForce=off  SenseTotalForceX=off  SenseTotalForceY=off  SenseTotalForceZ=off  SenseTotalTorque=off  SenseTotalTorqueX=off  SenseTotalTorqueY=off  SenseTotalTorqueZ=off  CompositeWrenchDir=FollowerOnBase  CompositeWrenchFrame=BaseFrame  EquilibriumPosition=0  EquilibriumPositionUnits=deg  SpringStiffness=IC.c_z  SpringStiffnessUnits=N*m/deg  DampingCoefficient=IC.d_z  DampingCoefficientUnits=N*m/(deg/s)  TorqueActuationMode=NoTorque  MotionActuationMode=ComputedMotion  SensePosition=on  SenseVelocity=on  SenseAcceleration=off  SenseTorqueForce=off  SenseLowerLimitTorqueForce=off  SenseUpperLimitTorqueForce=off  LowerLimitSpecify=on  LowerLimitBound=-IC.limit.phi_com  LowerLimitBoundUnits=rad  LowerLimitStiffness=1e4  LowerLimitStiffnessUnits=N*m/deg  LowerLimitDamping=10  LowerLimitDampingUnits=N*m/(deg/s)  LowerLimitTransitionRegionWidth=0.1  LowerLimitTransitionRegionWidthUnits=deg  UpperLimitSpecify=on  UpperLimitBound=IC.limit.phi_com  UpperLimitBoundUnits=rad  UpperLimitStiffness=1e4  UpperLimitStiffnessUnits=N*m/deg  UpperLimitDamping=10  UpperLimitDampingUnits=N*m/(deg/s)  UpperLimitTransitionRegionWidth=0.1  UpperLimitTransitionRegionWidthUnits=deg  PositionTargetSpecify=on  PositionTargetPriority=High  PositionTargetValue=IC.phi.com  PositionTargetValueUnits=rad  VelocityTargetSpecify=on  VelocityTargetPriority=High  VelocityTargetValue=IC.vphi.com  VelocityTargetValueUnits=rad/s
  Rigid Transform : sm_lib/Frames and Transforms/Rigid Transform  TranslationMethod=StandardAxis  TranslationStandardOffset=.5  TranslationLengthUnit=m  TranslationStandardAxis=+Z  TranslationCartesianOffset=[0 0 0]  TranslationROffset=0  TranslationROffsetUnits=m  TranslationZOffset=0  TranslationZOffsetUnits=m  TranslationThetaOffset=0  TranslationThetaOffsetUnits=deg  RotationMethod=None  RotationAngleUnits=deg  RotationStandardAxis=+Z  RotationAngle=0.0  RotationArbitraryAxis=[0 0 1]  FollAlignAxisA=+X  BaseAlignAxisA=+Y  FollAlignAxisB=+Y  BaseAlignAxisB=+Z  RotationSequenceAxes=FollowerAxes  RotationSequence=XYX  RotationSequenceAngles=[0 0 0]  RotationSequenceAnglesUnits=deg  RotationMatrix=[1 0 0; 0 1 0; 0 0 1]
  Rigid Transform1 : sm_lib/Frames and Transforms/Rigid Transform  TranslationMethod=StandardAxis  TranslationStandardOffset=.1  TranslationLengthUnit=m  TranslationStandardAxis=-Y  TranslationCartesianOffset=[0 0 0]  TranslationROffset=0  TranslationROffsetUnits=m  TranslationZOffset=0  TranslationZOffsetUnits=m  TranslationThetaOffset=0  TranslationThetaOffsetUnits=deg  RotationMethod=None  RotationAngleUnits=deg  RotationStandardAxis=+Z  RotationAngle=0.0  RotationArbitraryAxis=[0 0 1]  FollAlignAxisA=+X  BaseAlignAxisA=+Y  FollAlignAxisB=+Y  BaseAlignAxisB=+Z  RotationSequenceAxes=FollowerAxes  RotationSequence=XYX  RotationSequenceAngles=[0 0 0]  RotationSequenceAnglesUnits=deg  RotationMatrix=[1 0 0; 0 1 0; 0 0 1]
  World : PMIOPort  Side=Left
  Trunk : PMIOPort  Port=2  Side=Right
  tag scope: dx_com=global, dy_com=global, phi_com=global, phi_com_world=global, vphi_com=global, vphi_com_world=global, x_com=global, y_com=global
  wires:
  PS-Simulink Converter/1 -> [x_com]  "x_com"
  PS-Simulink Converter1/1 -> [dx_com]  "dx_com"
  PS-Simulink Converter3/1 -> [dy_com]  "dy_com"
  PS-Simulink Converter4/1 -> [phi_com]  "phi_com"
  PS-Simulink Converter2/1 -> [y_com]  "y_com"
  PS-Simulink Converter6/1 -> [phi_com_world]  "phi_com"
  PS-Simulink Converter5/1 -> [vphi_com]  "phi_com"
  PS-Simulink Converter7/1 -> [vphi_com_world]  "vphi_com_world"
  connections:
  Boom Rotation/LConn1 -- Boom Connector Coords/LConn1 -- World/RConn1
  Dummy boom connector/LConn1 -- Rigid Transform/LConn1 -- Boom Rotation/RConn1
  Dummy boom connector/RConn1 -- Pitch joint/LConn1
  Pitch joint/RConn1 -- Boom Connector Coords/RConn1 -- Trunk/RConn1
  PS-Simulink Converter5/LConn1 -- Pitch joint/RConn3
  Pitch joint/RConn2 -- PS-Simulink Converter4/LConn1
  Camera1/LConn1 -- Rigid Transform1/RConn1
  Rigid Transform1/LConn1 -- Rigid Transform/RConn1
  PS-Simulink Converter/LConn1 -- Boom Connector Coords/RConn4
  Boom Connector Coords/RConn5 -- PS-Simulink Converter2/LConn1
  Boom Connector Coords/RConn6 -- PS-Simulink Converter1/LConn1
  Boom Connector Coords/RConn7 -- PS-Simulink Converter3/LConn1
  Boom Connector Coords/RConn2 -- PS-Simulink Converter6/LConn1
  Boom Connector Coords/RConn3 -- PS-Simulink Converter7/LConn1
